simulink model "dynamic"  (R2025b)
settings: Solver=ode23t  StartTime=0.0  StopTime=100.0  MaxStep=1e-3  RelTol=1e-5
settings Model: Creator=violin

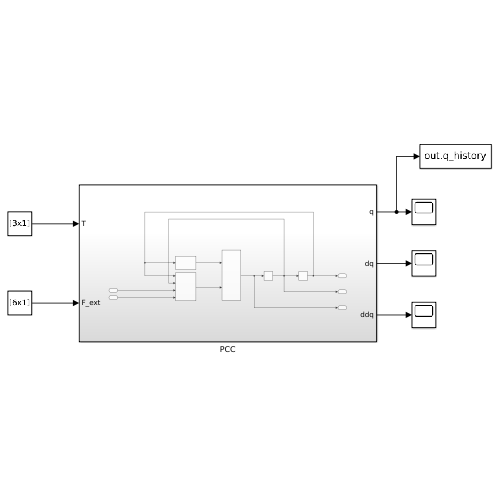
[thumbnail: Simulink's stored preview of the top-level diagram]
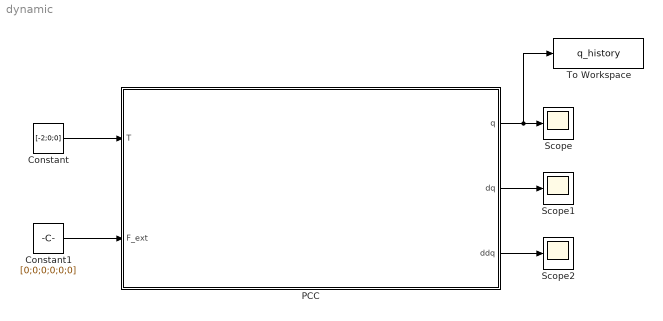
== system dynamic ==
  Constant : Constant  Value=[-2;0;0]
  Constant1 : Constant  Value=[0;0;0;0;0;0]
  PCC : Subsystem
  Scope : Scope
      settings: ActiveDisplayYMinimum=-0.073811965831007964  ActiveDisplayYMaximum=0.59923738312001884
  Scope1 : Scope
      settings: ActiveDisplayYMinimum=-1.2562951553581858  ActiveDisplayYMaximum=1.3493657939233712
  Scope2 : Scope
      settings: ActiveDisplayYMinimum=-3.5396008111253705  ActiveDisplayYMaximum=2.911379815977388  DataLoggingVariableName=ScopeData2
  To Workspace : ToWorkspace  VariableName=q_history  SampleTime=-1
  wires:
  Constant/1 -> PCC/1(T)
  Constant1/1 -> PCC/2(F_ext)
  PCC/1(q) -> To Workspace/1, Scope/1
  PCC/2(dq) -> Scope1/1
  PCC/3(ddq) -> Scope2/1

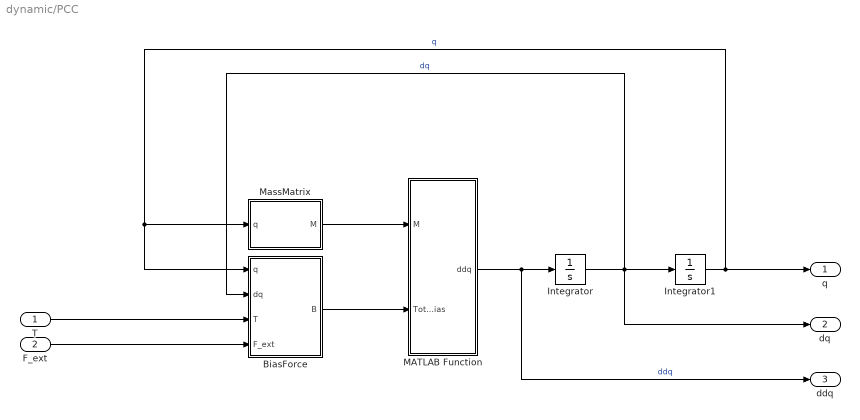
== system dynamic/PCC ==
  T : Inport
  F_ext : Inport  Port=2
  BiasForce : MATLAB Function  TreatAsAtomicUnit=on
  Integrator : Integrator  InitialCondition=zeros(6,1)
  Integrator1 : Integrator  InitialCondition=[0.1; 0; 0.5; 0.1; 0; 0.5]
  MATLAB Function : MATLAB Function  TreatAsAtomicUnit=on
  MassMatrix : MATLAB Function  TreatAsAtomicUnit=on
  q : Outport
  dq : Outport  Port=2
  ddq : Outport  Port=3
  wires:
  T/1 -> BiasForce/3(T)
  BiasForce/1(B) -> MATLAB Function/2(TotalBias)
  MassMatrix/1(M) -> MATLAB Function/1(M)
  MATLAB Function/1(ddq) -> ddq/1, Integrator/1  "ddq"
  Integrator1/1 -> q/1, BiasForce/1(q), MassMatrix/1(q)  "q"
  F_ext/1 -> BiasForce/4(F_ext)
  Integrator/1 -> dq/1, BiasForce/2(dq), Integrator1/1  "dq"

== matlab function dynamic/PCC/BiasForce ==
  data: q input; B output; dq input; T input; F_ext input
function B = fcn(q, dq, T, F_ext)

T1 = T(1); T2 = T(2); T3 = T(3);
fx = F_ext(1); fy = F_ext(2); fz = F_ext(3);
mx = F_ext(4); my = F_ext(5); mz = F_ext(6);
% B = get_BiasForce(q, dq, T1, T2, T3, fx, fy, fz, mx, my, mz);

GKForce = get_GKForce(q);
DampForce = get_DampForce(dq);
ExtForce = get_ExtForce(q, T1, T2, T3, fx, fy, fz, mx, my, mz);
B = GKForce+DampForce+ExtForce;

% EPSILON_THETA = 1e-3;
% 
% if q(1) < EPSILON_THETA
%     q(1) = EPSILON_THETA;
% end
% if q(4) < EPSILON_THETA
%     q(4) = EPSILON_THETA;
% end
% 
% CoriolisForce = get_Coriolis(q, dq);
% 
% B = B + CoriolisForce;

== matlab function dynamic/PCC/MassMatrix ==
  data: q input; M output
function M = fcn(q)

M = get_MassMatrix(q);

== matlab function dynamic/PCC/MATLAB Function ==
  data: M input; ddq output; TotalBias input
function ddq = Solver(M, TotalBias)

    M_stable = M + eye(size(M)) * 1e-5;

    ddq = M_stable \ (-TotalBias);
    
    limit = 1e3;
    ddq = max(min(ddq, limit), -limit);
end
